simulink model "Rozmyty_adaptacyjny"  (R2017b)
settings: Solver=ode1  StartTime=0.0  StopTime=10  FixedStep=0.0001  RelTol=1e-3
values from neighbouring files (symbols this model uses):
  Kd_adap = 50    [Dane_rozmyte.m]
  Kde1 = 0.02    [Dane_rozmyte.m]
  Kde2 = 0.05    [Dane_rozmyte.m]
  Ke1 = 1    [Dane_rozmyte.m]
  Ke2 = 1    [Dane_rozmyte.m]
  Kp_adap = 750    [Dane_rozmyte.m]
  ksi = 1    [Dane_rozmyte.m]
  Ku1 = 70    [Dane_rozmyte.m]
  Ku2 = 125    [Dane_rozmyte.m]
  omega = 30    [Dane_rozmyte.m]
  Te = 0.001    [Dane_rozmyte.m]
  Tm = 0.2    [Dane_rozmyte.m]
libraries: fuzblock x48
settings Model: Creator=kamil  LastModifiedBy=kamil

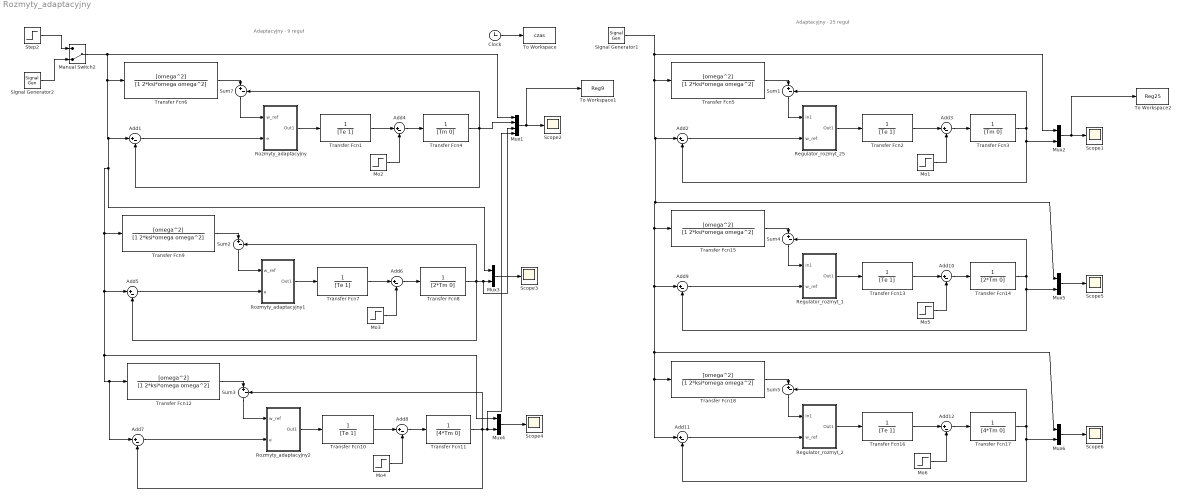
== system Rozmyty_adaptacyjny ==
  note: Adaptacyjny - 9 reguł
  note: Adaptacyjny - 25 reguł
  Add{1..12} (12 alike) : Sum  Inputs=|+-
  Clock : Clock
  Manual Switch2 : ManualSwitch  CurrentSetting=0
  Mo1 : Step  Time=3.5  After=0.5  SampleTime=0
  Mo2 : Step  Time=3  After=0.5  SampleTime=0
  Mo3 : Step  Time=3  After=0.5  SampleTime=0
  Mo4 : Step  Time=3  After=0.5  SampleTime=0
  Mo5 : Step  Time=3.5  After=0.5  SampleTime=0
  Mo6 : Step  Time=3.5  After=0.5  SampleTime=0
  Mux1 : Mux
  Mux{2..6} (5 alike) : Mux  Inputs=2
  Regulator_rozmyt_1 : Subsystem
  Regulator_rozmyt_2 : Subsystem
  Regulator_rozmyt_25 : Subsystem
  Rozmyty_adaptacyjny : Subsystem
  Rozmyty_adaptacyjny1 : Subsystem
  Rozmyty_adaptacyjny2 : Subsystem
  Scope{1..6} (6 alike) : Scope
  Signal Generator1 : SignalGenerator  WaveForm=square  Amplitude=0.25  Frequency=0.25
  Signal Generator2 : SignalGenerator  WaveForm=square  Amplitude=0.25  Frequency=0.25
  Step2 : Step  After=0.25  SampleTime=0
  Sum{1..5,7} (6 alike) : Sum  Inputs=|+-
  To Workspace : ToWorkspace  VariableName=czas  SampleTime=-1
  To Workspace1 : ToWorkspace  VariableName=Reg9  SampleTime=-1
  To Workspace2 : ToWorkspace  VariableName=Reg25  SampleTime=-1
  Transfer Fcn{1..2,7,10,13,16} (6 alike) : TransferFcn  Denominator=[Te 1]
  Transfer Fcn11 : TransferFcn  Denominator=[4*Tm 0]
  Transfer Fcn{5..6,9,12,15,18} (6 alike) : TransferFcn  Numerator=[omega^2]  Denominator=[1 2*ksi*omega omega^2]
  Transfer Fcn14 : TransferFcn  Denominator=[2*Tm 0]
  Transfer Fcn17 : TransferFcn  Denominator=[4*Tm 0]
  Transfer Fcn3 : TransferFcn  Denominator=[Tm 0]
  Transfer Fcn4 : TransferFcn  Denominator=[Tm 0]
  Transfer Fcn8 : TransferFcn  Denominator=[2*Tm 0]
  wires:
  Mo2/1 -> Add4/2
  Add4/1 -> Transfer Fcn4/1
  Transfer Fcn1/1 -> Add4/1
  Add1/1 -> Rozmyty_adaptacyjny/2(e)
  Transfer Fcn4/1 -> Sum7/2, Mux1/2, Add1/2
  Step2/1 -> Manual Switch2/1
  Signal Generator2/1 -> Manual Switch2/2
  Rozmyty_adaptacyjny/1(Out1) -> Transfer Fcn1/1
  Mux1/1 -> To Workspace1/1, Scope2/1
  Sum7/1 -> Rozmyty_adaptacyjny/1(w_ref)
  Transfer Fcn6/1 -> Sum7/1
  Clock/1 -> To Workspace/1
  Regulator_rozmyt_25/1(Out1) -> Transfer Fcn2/1
  Mo1/1 -> Add3/2
  Add3/1 -> Transfer Fcn3/1
  Transfer Fcn3/1 -> Mux2/2, Add2/2, Sum1/2
  Transfer Fcn2/1 -> Add3/1
  Sum1/1 -> Regulator_rozmyt_25/1(In1)
  Mux2/1 -> To Workspace2/1, Scope1/1
  Transfer Fcn5/1 -> Sum1/1
  Add2/1 -> Regulator_rozmyt_25/2(w_ref)
  Sum2/1 -> Rozmyty_adaptacyjny1/1(w_ref)
  Mux3/1 -> Scope3/1
  Transfer Fcn8/1 -> Sum2/2, Mux1/3, Mux3/2, Add5/2
  Transfer Fcn9/1 -> Sum2/1
  Mo3/1 -> Add6/2
  Add5/1 -> Rozmyty_adaptacyjny1/2(e)
  Add6/1 -> Transfer Fcn8/1
  Rozmyty_adaptacyjny1/1(Out1) -> Transfer Fcn7/1
  Transfer Fcn7/1 -> Add6/1
  Sum3/1 -> Rozmyty_adaptacyjny2/1(w_ref)
  Mux4/1 -> Scope4/1
  Transfer Fcn11/1 -> Sum3/2, Mux1/4, Mux4/2, Add7/2
  Transfer Fcn12/1 -> Sum3/1
  Manual Switch2/1 -> Transfer Fcn6/1, Transfer Fcn9/1, Mux4/1, Transfer Fcn12/1, Add7/1, Add5/1, Mux3/1, Add1/1, Mux1/1
  Mo4/1 -> Add8/2
  Add7/1 -> Rozmyty_adaptacyjny2/2(e)
  Add8/1 -> Transfer Fcn11/1
  Rozmyty_adaptacyjny2/1(Out1) -> Transfer Fcn10/1
  Transfer Fcn10/1 -> Add8/1
  Mux5/1 -> Scope5/1
  Add9/1 -> Regulator_rozmyt_1/2(w_ref)
  Transfer Fcn15/1 -> Sum4/1
  Transfer Fcn13/1 -> Add10/1
  Mo5/1 -> Add10/2
  Transfer Fcn14/1 -> Mux5/2, Add9/2, Sum4/2
  Add10/1 -> Transfer Fcn14/1
  Regulator_rozmyt_1/1(Out1) -> Transfer Fcn13/1
  Sum4/1 -> Regulator_rozmyt_1/1(In1)
  Signal Generator1/1 -> Transfer Fcn5/1, Transfer Fcn15/1, Transfer Fcn18/1, Add11/1, Mux6/1, Add9/1, Mux5/1, Add2/1, Mux2/1
  Mux6/1 -> Scope6/1
  Add11/1 -> Regulator_rozmyt_2/2(w_ref)
  Transfer Fcn18/1 -> Sum5/1
  Transfer Fcn16/1 -> Add12/1
  Mo6/1 -> Add12/2
  Transfer Fcn17/1 -> Mux6/2, Add11/2, Sum5/2
  Add12/1 -> Transfer Fcn17/1
  Regulator_rozmyt_2/1(Out1) -> Transfer Fcn16/1
  Sum5/1 -> Regulator_rozmyt_2/1(In1)

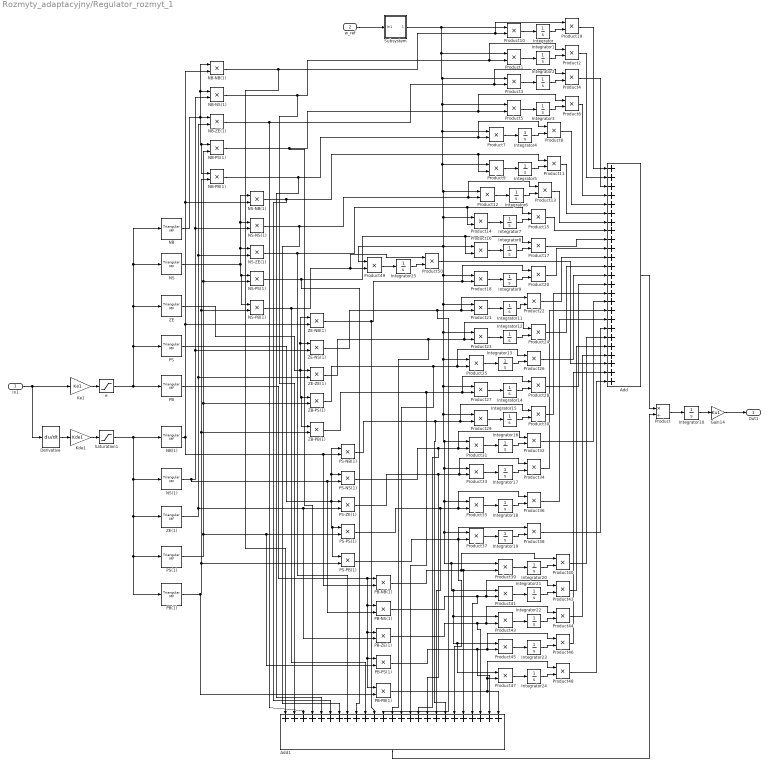
== system Rozmyty_adaptacyjny/Regulator_rozmyt_1 ==
  In1 : Inport
  w_ref : Inport  Port=2
  Add : Sum  Inputs=+++++++++++++++++++++++++
  Add1 : Sum  Inputs=+++++++++++++++++++++++++
  Derivative : Derivative
  Gain14 : Gain  Gain=Ku1
  Integrator{,1..25} (26 alike) : Integrator
  Kde1 : Gain  Gain=Kde1
  Ke1 : Gain  Gain=Ke1
  NB : fuzblock/Membership  Functions/Triangular MF  a=-1.5  b=-1  c=-0.5
      settings: SourceProductName=Fuzzy Logic Toolbox  SourceProductBaseCode=FL
  NB(1) : fuzblock/Membership  Functions/Triangular MF  a=-1.5  b=-1  c=-0.5
      settings: SourceProductName=Fuzzy Logic Toolbox  SourceProductBaseCode=FL
  NB-NB(1) : Product
  NB-NS(1) : Product
  NB-PB(1) : Product
  NB-PS(1) : Product
  NB-ZE(1) : Product
  NS : fuzblock/Membership  Functions/Triangular MF  a=-1  b=-0.5  c=0
      settings: SourceProductName=Fuzzy Logic Toolbox  SourceProductBaseCode=FL
  NS(1) : fuzblock/Membership  Functions/Triangular MF  a=-1  b=-0.5  c=0
      settings: SourceProductName=Fuzzy Logic Toolbox  SourceProductBaseCode=FL
  NS-NB(1) : Product
  NS-NS(1) : Product
  NS-PB(1) : Product
  NS-PS(1) : Product
  NS-ZE(1) : Product
  PB : fuzblock/Membership  Functions/Triangular MF  a=0.5  b=1  c=1.5
      settings: SourceProductName=Fuzzy Logic Toolbox  SourceProductBaseCode=FL
  PB(1) : fuzblock/Membership  Functions/Triangular MF  a=0.5  b=1  c=1.5
      settings: SourceProductName=Fuzzy Logic Toolbox  SourceProductBaseCode=FL
  PB-NB(1) : Product
  PB-NS(1) : Product
  PB-PB(1) : Product
  PB-PS(1) : Product
  PB-ZE(1) : Product
  PS : fuzblock/Membership  Functions/Triangular MF  a=0  b=0.5  c=1
      settings: SourceProductName=Fuzzy Logic Toolbox  SourceProductBaseCode=FL
  PS(1) : fuzblock/Membership  Functions/Triangular MF  a=0  b=0.5  c=1
      settings: SourceProductName=Fuzzy Logic Toolbox  SourceProductBaseCode=FL
  PS-NB(1) : Product
  PS-NS(1) : Product
  PS-PB(1) : Product
  PS-PS(1) : Product
  PS-ZE(1) : Product
  Product : Product  Inputs=*/
  Product{1..50} (50 alike) : Product
  Saturation1 : Saturate  UpperLimit=1  LowerLimit=-1
  Subsystem : Subsystem
  ZB-PB(1) : Product
  ZB-PS(1) : Product
  ZE : fuzblock/Membership  Functions/Triangular MF  a=-0.5  b=0  c=0.5
      settings: SourceProductName=Fuzzy Logic Toolbox  SourceProductBaseCode=FL
  ZE(1) : fuzblock/Membership  Functions/Triangular MF  a=-0.5  b=0  c=0.5
      settings: SourceProductName=Fuzzy Logic Toolbox  SourceProductBaseCode=FL
  ZE-NB(1) : Product
  ZE-NS(1) : Product
  ZE-ZE(1) : Product
  e : Saturate  UpperLimit=1  LowerLimit=-1
  Out1 : Outport
  wires:
  Ke1/1 -> e/1
  Kde1/1 -> Saturation1/1
  Derivative/1 -> Kde1/1
  In1/1 -> Derivative/1, Ke1/1
  e/1 -> PB/1, PS/1, NB/1, NS/1, ZE/1
  Saturation1/1 -> NB(1)/1, NS(1)/1, PB(1)/1, PS(1)/1, ZE(1)/1
  NS/1 -> NS-NB(1)/1, NS-NS(1)/1, NS-ZE(1)/1, NS-PB(1)/1, NS-PS(1)/1
  Add/1 -> Product/1
  Add1/1 -> Product/2
  Integrator10/1 -> Gain14/1
  Product/1 -> Integrator10/1
  Gain14/1 -> Out1/1
  NB/1 -> NB-NB(1)/1, NB-NS(1)/1, NB-ZE(1)/1, NB-PB(1)/1, NB-PS(1)/1
  ZE/1 -> ZE-NB(1)/1, ZE-NS(1)/1, ZE-ZE(1)/1, ZB-PB(1)/1, ZB-PS(1)/1
  PS/1 -> PS-NB(1)/1, PS-NS(1)/1, PS-ZE(1)/1, PS-PB(1)/1, PS-PS(1)/1
  PB/1 -> PB-ZE(1)/1, PB-PB(1)/1, PB-PS(1)/1, PB-NS(1)/1, PB-NB(1)/1
  NB(1)/1 -> PB-NB(1)/2, PS-NB(1)/2, ZE-NB(1)/2, NS-NB(1)/2, NB-NB(1)/2
  NS(1)/1 -> PB-NS(1)/2, PS-NS(1)/2, ZE-NS(1)/2, NS-NS(1)/2, NB-NS(1)/2
  ZE(1)/1 -> PB-ZE(1)/2, PS-ZE(1)/2, ZE-ZE(1)/2, NS-ZE(1)/2, NB-ZE(1)/2
  PS(1)/1 -> PB-PS(1)/2, PS-PS(1)/2, ZB-PS(1)/2, NS-PS(1)/2, NB-PS(1)/2
  PB(1)/1 -> PB-PB(1)/2, PS-PB(1)/2, ZB-PB(1)/2, NS-PB(1)/2, NB-PB(1)/2
  w_ref/1 -> Subsystem/1(In1)
  Product19/1 -> Add/1
  NB-NB(1)/1 -> Add1/1, Product10/2, Product19/1
  Product10/1 -> Integrator/1
  Subsystem/1(Out1) -> Product49/1, Product47/1, Product45/1, Product43/1, Product41/1, Product39/1, Product37/1, Product35/1, Product33/1, Product31/1, Product29/1, Product27/1, Product25/1, Product23/1, Product21/1, Product18/1, Product16/1, Product14/1, Product12/1, Product9/1, Product7/1, Product5/1, Product3/1, Product1/1, Product10/1
  Integrator/1 -> Product19/2
  Integrator1/1 -> Product2/2
  Product1/1 -> Integrator1/1
  NB-NS(1)/1 -> Add1/2, Product2/1, Product1/2
  Product2/1 -> Add/2
  Integrator2/1 -> Product4/2
  Product3/1 -> Integrator2/1
  NB-ZE(1)/1 -> Product4/1, Product3/2, Add1/3
  Product4/1 -> Add/3
  Integrator3/1 -> Product6/2
  Product5/1 -> Integrator3/1
  NB-PS(1)/1 -> Add1/4, Product6/1, Product5/2
  Product6/1 -> Add/4
  Integrator4/1 -> Product8/2
  Product7/1 -> Integrator4/1
  NB-PB(1)/1 -> Add1/5, Product8/1, Product7/2
  Product8/1 -> Add/5
  NS-NB(1)/1 -> Add1/6, Product9/2, Product11/1
  Product9/1 -> Integrator5/1
  Integrator5/1 -> Product11/2
  Product11/1 -> Add/6
  NS-NS(1)/1 -> Add1/7, Product13/1, Product12/2
  Product12/1 -> Integrator6/1
  Integrator6/1 -> Product13/2
  Product13/1 -> Add/7
  NS-ZE(1)/1 -> Add1/8, Product14/2, Product15/1
  Product14/1 -> Integrator7/1
  Integrator7/1 -> Product15/2
  Product15/1 -> Add/8
  NS-PS(1)/1 -> Add1/9, Product16/2, Product17/1
  Product16/1 -> Integrator8/1
  Integrator8/1 -> Product17/2
  Product17/1 -> Add/9
  ZE-NB(1)/1 -> Add1/11, Product18/2, Product20/1
  Product18/1 -> Integrator9/1
  Integrator9/1 -> Product20/2
  Product20/1 -> Add/10
  ZE-NS(1)/1 -> Add1/12, Product22/1, Product21/2
  Product21/1 -> Integrator11/1
  Integrator11/1 -> Product22/2
  Product22/1 -> Add/11
  ZE-ZE(1)/1 -> Add1/13, Product24/1, Product23/2
  Product23/1 -> Integrator12/1
  Integrator12/1 -> Product24/2
  Product24/1 -> Add/12
  ZB-PS(1)/1 -> Add1/14, Product26/1, Product25/2
  Product25/1 -> Integrator13/1
  Integrator13/1 -> Product26/2
  Product26/1 -> Add/13
  ZB-PB(1)/1 -> Add1/15, Product28/1, Product27/2
  Product27/1 -> Integrator14/1
  Integrator14/1 -> Product28/2
  Product28/1 -> Add/14
  PS-NB(1)/1 -> Add1/19, Product29/2, Product30/1
  Product29/1 -> Integrator15/1
  Integrator15/1 -> Product30/2
  PS-NS(1)/1 -> Add1/16, Product32/1, Product31/2
  Product31/1 -> Integrator16/1
  Integrator16/1 -> Product32/2
  PS-ZE(1)/1 -> Add1/17, Product34/1, Product33/2
  Product33/1 -> Integrator17/1
  Integrator17/1 -> Product34/2
  PS-PS(1)/1 -> Add1/18, Product36/1, Product35/2
  Product35/1 -> Integrator18/1
  Integrator18/1 -> Product36/2
  PS-PB(1)/1 -> Add1/20, Product37/2, Product38/1
  Product37/1 -> Integrator19/1
  Integrator19/1 -> Product38/2
  Product39/1 -> Integrator20/1
  Integrator20/1 -> Product40/2
  PB-NB(1)/1 -> Add1/21, Product39/2, Product40/1
  PB-NS(1)/1 -> Add1/22, Product42/1, Product41/2
  Product41/1 -> Integrator21/1
  Integrator21/1 -> Product42/2
  PB-ZE(1)/1 -> Add1/23, Product44/1, Product43/2
  Product43/1 -> Integrator22/1
  Integrator22/1 -> Product44/2
  PB-PS(1)/1 -> Add1/24, Product46/1, Product45/2
  Product45/1 -> Integrator23/1
  Integrator23/1 -> Product46/2
  PB-PB(1)/1 -> Add1/25, Product48/1, Product47/2
  Product47/1 -> Integrator24/1
  Integrator24/1 -> Product48/2
  Product30/1 -> Add/15
  Product32/1 -> Add/16
  Product34/1 -> Add/17
  Product36/1 -> Add/18
  Product38/1 -> Add/19
  Product40/1 -> Add/20
  Product42/1 -> Add/21
  Product44/1 -> Add/22
  Product46/1 -> Add/24
  Product48/1 -> Add/25
  NS-PB(1)/1 -> Add1/10, Product50/1, Product49/2
  Product49/1 -> Integrator25/1
  Integrator25/1 -> Product50/2
  Product50/1 -> Add/23

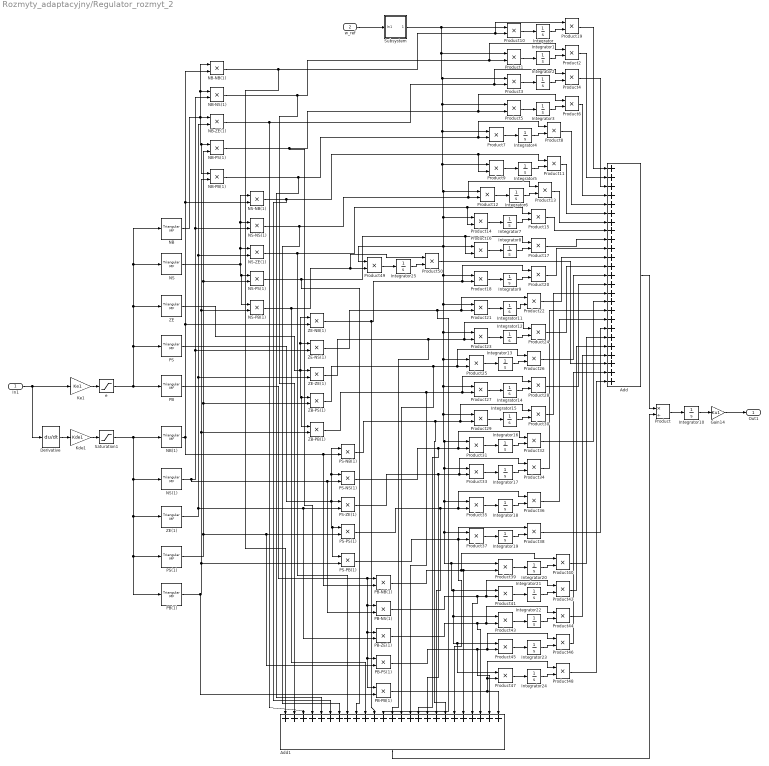
== system Rozmyty_adaptacyjny/Regulator_rozmyt_2 ==
  In1 : Inport
  w_ref : Inport  Port=2
  Add : Sum  Inputs=+++++++++++++++++++++++++
  Add1 : Sum  Inputs=+++++++++++++++++++++++++
  Derivative : Derivative
  Gain14 : Gain  Gain=Ku1
  Integrator{,1..25} (26 alike) : Integrator
  Kde1 : Gain  Gain=Kde1
  Ke1 : Gain  Gain=Ke1
  NB : fuzblock/Membership  Functions/Triangular MF  a=-1.5  b=-1  c=-0.5
      settings: SourceProductName=Fuzzy Logic Toolbox  SourceProductBaseCode=FL
  NB(1) : fuzblock/Membership  Functions/Triangular MF  a=-1.5  b=-1  c=-0.5
      settings: SourceProductName=Fuzzy Logic Toolbox  SourceProductBaseCode=FL
  NB-NB(1) : Product
  NB-NS(1) : Product
  NB-PB(1) : Product
  NB-PS(1) : Product
  NB-ZE(1) : Product
  NS : fuzblock/Membership  Functions/Triangular MF  a=-1  b=-0.5  c=0
      settings: SourceProductName=Fuzzy Logic Toolbox  SourceProductBaseCode=FL
  NS(1) : fuzblock/Membership  Functions/Triangular MF  a=-1  b=-0.5  c=0
      settings: SourceProductName=Fuzzy Logic Toolbox  SourceProductBaseCode=FL
  NS-NB(1) : Product
  NS-NS(1) : Product
  NS-PB(1) : Product
  NS-PS(1) : Product
  NS-ZE(1) : Product
  PB : fuzblock/Membership  Functions/Triangular MF  a=0.5  b=1  c=1.5
      settings: SourceProductName=Fuzzy Logic Toolbox  SourceProductBaseCode=FL
  PB(1) : fuzblock/Membership  Functions/Triangular MF  a=0.5  b=1  c=1.5
      settings: SourceProductName=Fuzzy Logic Toolbox  SourceProductBaseCode=FL
  PB-NB(1) : Product
  PB-NS(1) : Product
  PB-PB(1) : Product
  PB-PS(1) : Product
  PB-ZE(1) : Product
  PS : fuzblock/Membership  Functions/Triangular MF  a=0  b=0.5  c=1
      settings: SourceProductName=Fuzzy Logic Toolbox  SourceProductBaseCode=FL
  PS(1) : fuzblock/Membership  Functions/Triangular MF  a=0  b=0.5  c=1
      settings: SourceProductName=Fuzzy Logic Toolbox  SourceProductBaseCode=FL
  PS-NB(1) : Product
  PS-NS(1) : Product
  PS-PB(1) : Product
  PS-PS(1) : Product
  PS-ZE(1) : Product
  Product : Product  Inputs=*/
  Product{1..50} (50 alike) : Product
  Saturation1 : Saturate  UpperLimit=1  LowerLimit=-1
  Subsystem : Subsystem
  ZB-PB(1) : Product
  ZB-PS(1) : Product
  ZE : fuzblock/Membership  Functions/Triangular MF  a=-0.5  b=0  c=0.5
      settings: SourceProductName=Fuzzy Logic Toolbox  SourceProductBaseCode=FL
  ZE(1) : fuzblock/Membership  Functions/Triangular MF  a=-0.5  b=0  c=0.5
      settings: SourceProductName=Fuzzy Logic Toolbox  SourceProductBaseCode=FL
  ZE-NB(1) : Product
  ZE-NS(1) : Product
  ZE-ZE(1) : Product
  e : Saturate  UpperLimit=1  LowerLimit=-1
  Out1 : Outport
  wires:
  Ke1/1 -> e/1
  Kde1/1 -> Saturation1/1
  Derivative/1 -> Kde1/1
  In1/1 -> Derivative/1, Ke1/1
  e/1 -> PB/1, PS/1, NB/1, NS/1, ZE/1
  Saturation1/1 -> NB(1)/1, NS(1)/1, PB(1)/1, PS(1)/1, ZE(1)/1
  NS/1 -> NS-NB(1)/1, NS-NS(1)/1, NS-ZE(1)/1, NS-PB(1)/1, NS-PS(1)/1
  Add/1 -> Product/1
  Add1/1 -> Product/2
  Integrator10/1 -> Gain14/1
  Product/1 -> Integrator10/1
  Gain14/1 -> Out1/1
  NB/1 -> NB-NB(1)/1, NB-NS(1)/1, NB-ZE(1)/1, NB-PB(1)/1, NB-PS(1)/1
  ZE/1 -> ZE-NB(1)/1, ZE-NS(1)/1, ZE-ZE(1)/1, ZB-PB(1)/1, ZB-PS(1)/1
  PS/1 -> PS-NB(1)/1, PS-NS(1)/1, PS-ZE(1)/1, PS-PB(1)/1, PS-PS(1)/1
  PB/1 -> PB-ZE(1)/1, PB-PB(1)/1, PB-PS(1)/1, PB-NS(1)/1, PB-NB(1)/1
  NB(1)/1 -> PB-NB(1)/2, PS-NB(1)/2, ZE-NB(1)/2, NS-NB(1)/2, NB-NB(1)/2
  NS(1)/1 -> PB-NS(1)/2, PS-NS(1)/2, ZE-NS(1)/2, NS-NS(1)/2, NB-NS(1)/2
  ZE(1)/1 -> PB-ZE(1)/2, PS-ZE(1)/2, ZE-ZE(1)/2, NS-ZE(1)/2, NB-ZE(1)/2
  PS(1)/1 -> PB-PS(1)/2, PS-PS(1)/2, ZB-PS(1)/2, NS-PS(1)/2, NB-PS(1)/2
  PB(1)/1 -> PB-PB(1)/2, PS-PB(1)/2, ZB-PB(1)/2, NS-PB(1)/2, NB-PB(1)/2
  w_ref/1 -> Subsystem/1(In1)
  Product19/1 -> Add/1
  NB-NB(1)/1 -> Add1/1, Product10/2, Product19/1
  Product10/1 -> Integrator/1
  Subsystem/1(Out1) -> Product49/1, Product47/1, Product45/1, Product43/1, Product41/1, Product39/1, Product37/1, Product35/1, Product33/1, Product31/1, Product29/1, Product27/1, Product25/1, Product23/1, Product21/1, Product18/1, Product16/1, Product14/1, Product12/1, Product9/1, Product7/1, Product5/1, Product3/1, Product1/1, Product10/1
  Integrator/1 -> Product19/2
  Integrator1/1 -> Product2/2
  Product1/1 -> Integrator1/1
  NB-NS(1)/1 -> Add1/2, Product2/1, Product1/2
  Product2/1 -> Add/2
  Integrator2/1 -> Product4/2
  Product3/1 -> Integrator2/1
  NB-ZE(1)/1 -> Product4/1, Product3/2, Add1/3
  Product4/1 -> Add/3
  Integrator3/1 -> Product6/2
  Product5/1 -> Integrator3/1
  NB-PS(1)/1 -> Add1/4, Product6/1, Product5/2
  Product6/1 -> Add/4
  Integrator4/1 -> Product8/2
  Product7/1 -> Integrator4/1
  NB-PB(1)/1 -> Add1/5, Product8/1, Product7/2
  Product8/1 -> Add/5
  NS-NB(1)/1 -> Add1/6, Product9/2, Product11/1
  Product9/1 -> Integrator5/1
  Integrator5/1 -> Product11/2
  Product11/1 -> Add/6
  NS-NS(1)/1 -> Add1/7, Product13/1, Product12/2
  Product12/1 -> Integrator6/1
  Integrator6/1 -> Product13/2
  Product13/1 -> Add/7
  NS-ZE(1)/1 -> Add1/8, Product14/2, Product15/1
  Product14/1 -> Integrator7/1
  Integrator7/1 -> Product15/2
  Product15/1 -> Add/8
  NS-PS(1)/1 -> Add1/9, Product16/2, Product17/1
  Product16/1 -> Integrator8/1
  Integrator8/1 -> Product17/2
  Product17/1 -> Add/9
  ZE-NB(1)/1 -> Add1/11, Product18/2, Product20/1
  Product18/1 -> Integrator9/1
  Integrator9/1 -> Product20/2
  Product20/1 -> Add/10
  ZE-NS(1)/1 -> Add1/12, Product22/1, Product21/2
  Product21/1 -> Integrator11/1
  Integrator11/1 -> Product22/2
  Product22/1 -> Add/11
  ZE-ZE(1)/1 -> Add1/13, Product24/1, Product23/2
  Product23/1 -> Integrator12/1
  Integrator12/1 -> Product24/2
  Product24/1 -> Add/12
  ZB-PS(1)/1 -> Add1/14, Product26/1, Product25/2
  Product25/1 -> Integrator13/1
  Integrator13/1 -> Product26/2
  Product26/1 -> Add/13
  ZB-PB(1)/1 -> Add1/15, Product28/1, Product27/2
  Product27/1 -> Integrator14/1
  Integrator14/1 -> Product28/2
  Product28/1 -> Add/14
  PS-NB(1)/1 -> Add1/19, Product29/2, Product30/1
  Product29/1 -> Integrator15/1
  Integrator15/1 -> Product30/2
  PS-NS(1)/1 -> Add1/16, Product32/1, Product31/2
  Product31/1 -> Integrator16/1
  Integrator16/1 -> Product32/2
  PS-ZE(1)/1 -> Add1/17, Product34/1, Product33/2
  Product33/1 -> Integrator17/1
  Integrator17/1 -> Product34/2
  PS-PS(1)/1 -> Add1/18, Product36/1, Product35/2
  Product35/1 -> Integrator18/1
  Integrator18/1 -> Product36/2
  PS-PB(1)/1 -> Add1/20, Product37/2, Product38/1
  Product37/1 -> Integrator19/1
  Integrator19/1 -> Product38/2
  Product39/1 -> Integrator20/1
  Integrator20/1 -> Product40/2
  PB-NB(1)/1 -> Add1/21, Product39/2, Product40/1
  PB-NS(1)/1 -> Add1/22, Product42/1, Product41/2
  Product41/1 -> Integrator21/1
  Integrator21/1 -> Product42/2
  PB-ZE(1)/1 -> Add1/23, Product44/1, Product43/2
  Product43/1 -> Integrator22/1
  Integrator22/1 -> Product44/2
  PB-PS(1)/1 -> Add1/24, Product46/1, Product45/2
  Product45/1 -> Integrator23/1
  Integrator23/1 -> Product46/2
  PB-PB(1)/1 -> Add1/25, Product48/1, Product47/2
  Product47/1 -> Integrator24/1
  Integrator24/1 -> Product48/2
  Product30/1 -> Add/15
  Product32/1 -> Add/16
  Product34/1 -> Add/17
  Product36/1 -> Add/18
  Product38/1 -> Add/19
  Product40/1 -> Add/20
  Product42/1 -> Add/21
  Product44/1 -> Add/22
  Product46/1 -> Add/24
  Product48/1 -> Add/25
  NS-PB(1)/1 -> Add1/10, Product50/1, Product49/2
  Product49/1 -> Integrator25/1
  Integrator25/1 -> Product50/2
  Product50/1 -> Add/23

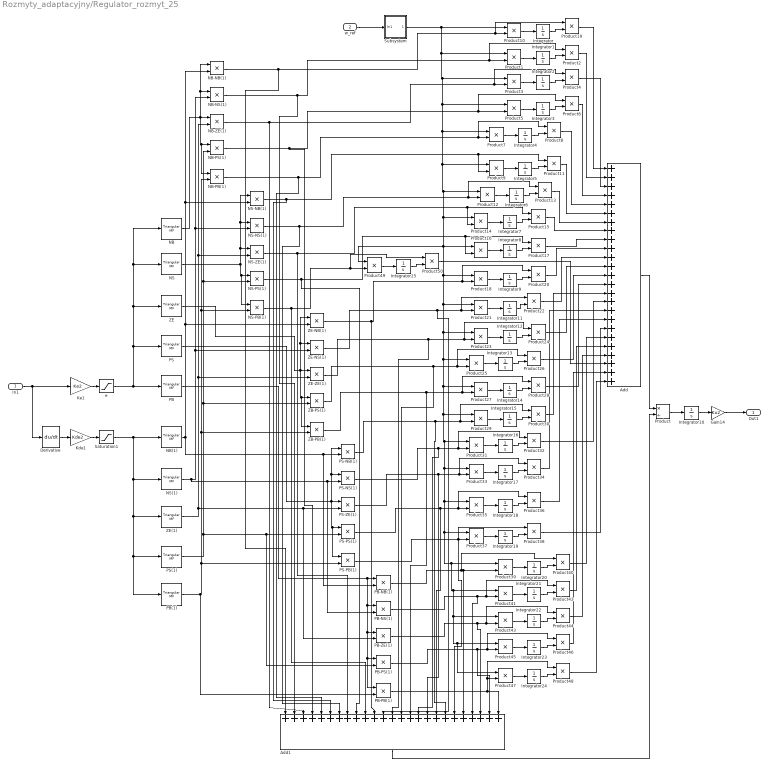
== system Rozmyty_adaptacyjny/Regulator_rozmyt_25 ==
  In1 : Inport
  w_ref : Inport  Port=2
  Add : Sum  Inputs=+++++++++++++++++++++++++
  Add1 : Sum  Inputs=+++++++++++++++++++++++++
  Derivative : Derivative
  Gain14 : Gain  Gain=Ku2
  Integrator{,1..25} (26 alike) : Integrator
  Kde1 : Gain  Gain=Kde2
  Ke1 : Gain  Gain=Ke2
  NB : fuzblock/Membership  Functions/Triangular MF  a=-1.5  b=-1  c=-0.5
      settings: SourceProductName=Fuzzy Logic Toolbox  SourceProductBaseCode=FL
  NB(1) : fuzblock/Membership  Functions/Triangular MF  a=-1.5  b=-1  c=-0.5
      settings: SourceProductName=Fuzzy Logic Toolbox  SourceProductBaseCode=FL
  NB-NB(1) : Product
  NB-NS(1) : Product
  NB-PB(1) : Product
  NB-PS(1) : Product
  NB-ZE(1) : Product
  NS : fuzblock/Membership  Functions/Triangular MF  a=-1  b=-0.5  c=0
      settings: SourceProductName=Fuzzy Logic Toolbox  SourceProductBaseCode=FL
  NS(1) : fuzblock/Membership  Functions/Triangular MF  a=-1  b=-0.5  c=0
      settings: SourceProductName=Fuzzy Logic Toolbox  SourceProductBaseCode=FL
  NS-NB(1) : Product
  NS-NS(1) : Product
  NS-PB(1) : Product
  NS-PS(1) : Product
  NS-ZE(1) : Product
  PB : fuzblock/Membership  Functions/Triangular MF  a=0.5  b=1  c=1.5
      settings: SourceProductName=Fuzzy Logic Toolbox  SourceProductBaseCode=FL
  PB(1) : fuzblock/Membership  Functions/Triangular MF  a=0.5  b=1  c=1.5
      settings: SourceProductName=Fuzzy Logic Toolbox  SourceProductBaseCode=FL
  PB-NB(1) : Product
  PB-NS(1) : Product
  PB-PB(1) : Product
  PB-PS(1) : Product
  PB-ZE(1) : Product
  PS : fuzblock/Membership  Functions/Triangular MF  a=0  b=0.5  c=1
      settings: SourceProductName=Fuzzy Logic Toolbox  SourceProductBaseCode=FL
  PS(1) : fuzblock/Membership  Functions/Triangular MF  a=0  b=0.5  c=1
      settings: SourceProductName=Fuzzy Logic Toolbox  SourceProductBaseCode=FL
  PS-NB(1) : Product
  PS-NS(1) : Product
  PS-PB(1) : Product
  PS-PS(1) : Product
  PS-ZE(1) : Product
  Product : Product  Inputs=*/
  Product{1..50} (50 alike) : Product
  Saturation1 : Saturate  UpperLimit=1  LowerLimit=-1
  Subsystem : Subsystem
  ZB-PB(1) : Product
  ZB-PS(1) : Product
  ZE : fuzblock/Membership  Functions/Triangular MF  a=-0.5  b=0  c=0.5
      settings: SourceProductName=Fuzzy Logic Toolbox  SourceProductBaseCode=FL
  ZE(1) : fuzblock/Membership  Functions/Triangular MF  a=-0.5  b=0  c=0.5
      settings: SourceProductName=Fuzzy Logic Toolbox  SourceProductBaseCode=FL
  ZE-NB(1) : Product
  ZE-NS(1) : Product
  ZE-ZE(1) : Product
  e : Saturate  UpperLimit=1  LowerLimit=-1
  Out1 : Outport
  wires:
  Ke1/1 -> e/1
  Kde1/1 -> Saturation1/1
  Derivative/1 -> Kde1/1
  In1/1 -> Derivative/1, Ke1/1
  e/1 -> PB/1, PS/1, NB/1, NS/1, ZE/1
  Saturation1/1 -> NB(1)/1, NS(1)/1, PB(1)/1, PS(1)/1, ZE(1)/1
  NS/1 -> NS-NB(1)/1, NS-NS(1)/1, NS-ZE(1)/1, NS-PB(1)/1, NS-PS(1)/1
  Add/1 -> Product/1
  Add1/1 -> Product/2
  Integrator10/1 -> Gain14/1
  Product/1 -> Integrator10/1
  Gain14/1 -> Out1/1
  NB/1 -> NB-NB(1)/1, NB-NS(1)/1, NB-ZE(1)/1, NB-PB(1)/1, NB-PS(1)/1
  ZE/1 -> ZE-NB(1)/1, ZE-NS(1)/1, ZE-ZE(1)/1, ZB-PB(1)/1, ZB-PS(1)/1
  PS/1 -> PS-NB(1)/1, PS-NS(1)/1, PS-ZE(1)/1, PS-PB(1)/1, PS-PS(1)/1
  PB/1 -> PB-ZE(1)/1, PB-PB(1)/1, PB-PS(1)/1, PB-NS(1)/1, PB-NB(1)/1
  NB(1)/1 -> PB-NB(1)/2, PS-NB(1)/2, ZE-NB(1)/2, NS-NB(1)/2, NB-NB(1)/2
  NS(1)/1 -> PB-NS(1)/2, PS-NS(1)/2, ZE-NS(1)/2, NS-NS(1)/2, NB-NS(1)/2
  ZE(1)/1 -> PB-ZE(1)/2, PS-ZE(1)/2, ZE-ZE(1)/2, NS-ZE(1)/2, NB-ZE(1)/2
  PS(1)/1 -> PB-PS(1)/2, PS-PS(1)/2, ZB-PS(1)/2, NS-PS(1)/2, NB-PS(1)/2
  PB(1)/1 -> PB-PB(1)/2, PS-PB(1)/2, ZB-PB(1)/2, NS-PB(1)/2, NB-PB(1)/2
  w_ref/1 -> Subsystem/1(In1)
  Product19/1 -> Add/1
  NB-NB(1)/1 -> Add1/1, Product10/2, Product19/1
  Product10/1 -> Integrator/1
  Subsystem/1(Out1) -> Product49/1, Product47/1, Product45/1, Product43/1, Product41/1, Product39/1, Product37/1, Product35/1, Product33/1, Product31/1, Product29/1, Product27/1, Product25/1, Product23/1, Product21/1, Product18/1, Product16/1, Product14/1, Product12/1, Product9/1, Product7/1, Product5/1, Product3/1, Product1/1, Product10/1
  Integrator/1 -> Product19/2
  Integrator1/1 -> Product2/2
  Product1/1 -> Integrator1/1
  NB-NS(1)/1 -> Add1/2, Product2/1, Product1/2
  Product2/1 -> Add/2
  Integrator2/1 -> Product4/2
  Product3/1 -> Integrator2/1
  NB-ZE(1)/1 -> Product4/1, Product3/2, Add1/3
  Product4/1 -> Add/3
  Integrator3/1 -> Product6/2
  Product5/1 -> Integrator3/1
  NB-PS(1)/1 -> Add1/4, Product6/1, Product5/2
  Product6/1 -> Add/4
  Integrator4/1 -> Product8/2
  Product7/1 -> Integrator4/1
  NB-PB(1)/1 -> Add1/5, Product8/1, Product7/2
  Product8/1 -> Add/5
  NS-NB(1)/1 -> Add1/6, Product9/2, Product11/1
  Product9/1 -> Integrator5/1
  Integrator5/1 -> Product11/2
  Product11/1 -> Add/6
  NS-NS(1)/1 -> Add1/7, Product13/1, Product12/2
  Product12/1 -> Integrator6/1
  Integrator6/1 -> Product13/2
  Product13/1 -> Add/7
  NS-ZE(1)/1 -> Add1/8, Product14/2, Product15/1
  Product14/1 -> Integrator7/1
  Integrator7/1 -> Product15/2
  Product15/1 -> Add/8
  NS-PS(1)/1 -> Add1/9, Product16/2, Product17/1
  Product16/1 -> Integrator8/1
  Integrator8/1 -> Product17/2
  Product17/1 -> Add/9
  ZE-NB(1)/1 -> Add1/11, Product18/2, Product20/1
  Product18/1 -> Integrator9/1
  Integrator9/1 -> Product20/2
  Product20/1 -> Add/10
  ZE-NS(1)/1 -> Add1/12, Product22/1, Product21/2
  Product21/1 -> Integrator11/1
  Integrator11/1 -> Product22/2
  Product22/1 -> Add/11
  ZE-ZE(1)/1 -> Add1/13, Product24/1, Product23/2
  Product23/1 -> Integrator12/1
  Integrator12/1 -> Product24/2
  Product24/1 -> Add/12
  ZB-PS(1)/1 -> Add1/14, Product26/1, Product25/2
  Product25/1 -> Integrator13/1
  Integrator13/1 -> Product26/2
  Product26/1 -> Add/13
  ZB-PB(1)/1 -> Add1/15, Product28/1, Product27/2
  Product27/1 -> Integrator14/1
  Integrator14/1 -> Product28/2
  Product28/1 -> Add/14
  PS-NB(1)/1 -> Add1/19, Product29/2, Product30/1
  Product29/1 -> Integrator15/1
  Integrator15/1 -> Product30/2
  PS-NS(1)/1 -> Add1/16, Product32/1, Product31/2
  Product31/1 -> Integrator16/1
  Integrator16/1 -> Product32/2
  PS-ZE(1)/1 -> Add1/17, Product34/1, Product33/2
  Product33/1 -> Integrator17/1
  Integrator17/1 -> Product34/2
  PS-PS(1)/1 -> Add1/18, Product36/1, Product35/2
  Product35/1 -> Integrator18/1
  Integrator18/1 -> Product36/2
  PS-PB(1)/1 -> Add1/20, Product37/2, Product38/1
  Product37/1 -> Integrator19/1
  Integrator19/1 -> Product38/2
  Product39/1 -> Integrator20/1
  Integrator20/1 -> Product40/2
  PB-NB(1)/1 -> Add1/21, Product39/2, Product40/1
  PB-NS(1)/1 -> Add1/22, Product42/1, Product41/2
  Product41/1 -> Integrator21/1
  Integrator21/1 -> Product42/2
  PB-ZE(1)/1 -> Add1/23, Product44/1, Product43/2
  Product43/1 -> Integrator22/1
  Integrator22/1 -> Product44/2
  PB-PS(1)/1 -> Add1/24, Product46/1, Product45/2
  Product45/1 -> Integrator23/1
  Integrator23/1 -> Product46/2
  PB-PB(1)/1 -> Add1/25, Product48/1, Product47/2
  Product47/1 -> Integrator24/1
  Integrator24/1 -> Product48/2
  Product30/1 -> Add/15
  Product32/1 -> Add/16
  Product34/1 -> Add/17
  Product36/1 -> Add/18
  Product38/1 -> Add/19
  Product40/1 -> Add/20
  Product42/1 -> Add/21
  Product44/1 -> Add/22
  Product46/1 -> Add/24
  Product48/1 -> Add/25
  NS-PB(1)/1 -> Add1/10, Product50/1, Product49/2
  Product49/1 -> Integrator25/1
  Integrator25/1 -> Product50/2
  Product50/1 -> Add/23

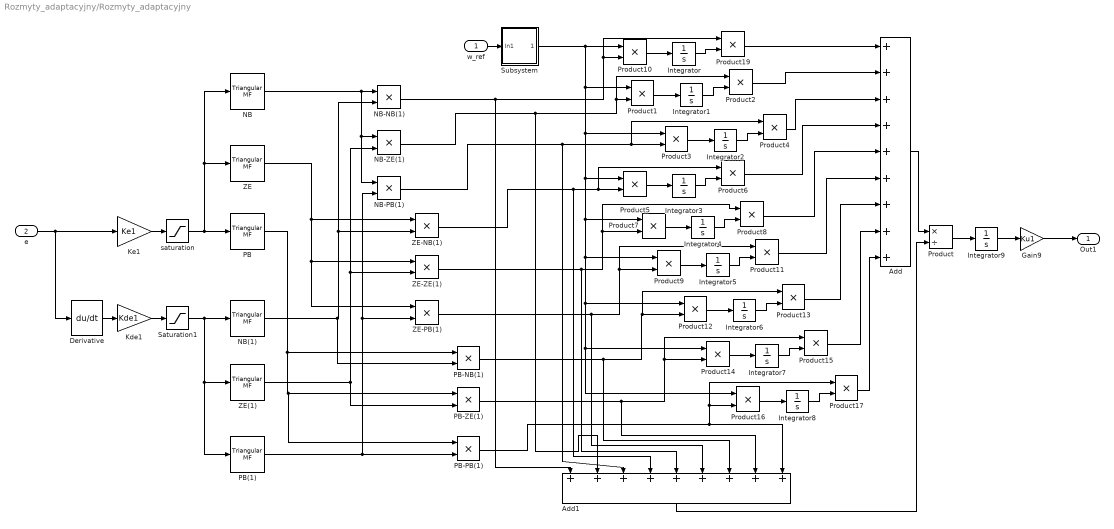
== system Rozmyty_adaptacyjny/Rozmyty_adaptacyjny ==
  w_ref : Inport
  e : Inport  Port=2
  Add : Sum  Inputs=+++++++++
  Add1 : Sum  Inputs=+++++++++
  Derivative : Derivative
  Gain9 : Gain  Gain=Ku1
  Integrator{,1..9} (10 alike) : Integrator
  Kde1 : Gain  Gain=Kde1
  Ke1 : Gain  Gain=Ke1
  NB : fuzblock/Membership  Functions/Triangular MF  a=-2  b=-1  c=0
      settings: SourceProductName=Fuzzy Logic Toolbox  SourceProductBaseCode=FL
  NB(1) : fuzblock/Membership  Functions/Triangular MF  a=-2  b=-1  c=0
      settings: SourceProductName=Fuzzy Logic Toolbox  SourceProductBaseCode=FL
  NB-NB(1) : Product
  NB-PB(1) : Product
  NB-ZE(1) : Product
  PB : fuzblock/Membership  Functions/Triangular MF  a=0  b=1  c=2
      settings: SourceProductName=Fuzzy Logic Toolbox  SourceProductBaseCode=FL
  PB(1) : fuzblock/Membership  Functions/Triangular MF  a=0  b=1  c=2
      settings: SourceProductName=Fuzzy Logic Toolbox  SourceProductBaseCode=FL
  PB-NB(1) : Product
  PB-PB(1) : Product
  PB-ZE(1) : Product
  Product : Product  Inputs=*/
  Product{1..17,19} (18 alike) : Product
  Saturation1 : Saturate  UpperLimit=1  LowerLimit=-1
  Subsystem : Subsystem
  ZE : fuzblock/Membership  Functions/Triangular MF  a=-1  b=0  c=1
      settings: SourceProductName=Fuzzy Logic Toolbox  SourceProductBaseCode=FL
  ZE(1) : fuzblock/Membership  Functions/Triangular MF  a=-1  b=0  c=1
      settings: SourceProductName=Fuzzy Logic Toolbox  SourceProductBaseCode=FL
  ZE-NB(1) : Product
  ZE-PB(1) : Product
  ZE-ZE(1) : Product
  saturation : Saturate  UpperLimit=1  LowerLimit=-1
  Out1 : Outport
  wires:
  Ke1/1 -> saturation/1
  Kde1/1 -> Saturation1/1
  Derivative/1 -> Kde1/1
  e/1 -> Derivative/1, Ke1/1
  saturation/1 -> PB/1, NB/1, ZE/1
  Saturation1/1 -> PB(1)/1, ZE(1)/1, NB(1)/1
  NB/1 -> NB-ZE(1)/1, NB-PB(1)/1, NB-NB(1)/1
  NB(1)/1 -> PB-NB(1)/2, NB-NB(1)/2, ZE-NB(1)/2
  ZE(1)/1 -> PB-ZE(1)/2, NB-ZE(1)/2, ZE-ZE(1)/2
  PB(1)/1 -> NB-PB(1)/2, ZE-PB(1)/2, PB-PB(1)/2
  ZE/1 -> ZE-NB(1)/1, ZE-ZE(1)/1, ZE-PB(1)/1
  PB/1 -> PB-NB(1)/1, PB-PB(1)/1, PB-ZE(1)/1
  Add/1 -> Product/1
  Add1/1 -> Product/2
  Integrator9/1 -> Gain9/1
  Product/1 -> Integrator9/1
  Gain9/1 -> Out1/1
  Product10/1 -> Integrator/1
  Integrator/1 -> Product19/2
  Product19/1 -> Add/1
  w_ref/1 -> Subsystem/1(In1)
  Product1/1 -> Integrator1/1
  NB-ZE(1)/1 -> Add1/2, Product1/2, Product2/1
  NB-NB(1)/1 -> Product10/2, Product19/1, Add1/1
  Integrator1/1 -> Product2/2
  Product2/1 -> Add/2
  Product3/1 -> Integrator2/1
  NB-PB(1)/1 -> Add1/3, Product4/1, Product3/2
  Integrator2/1 -> Product4/2
  Product4/1 -> Add/3
  Product5/1 -> Integrator3/1
  ZE-NB(1)/1 -> Add1/4, Product6/1, Product5/2
  Integrator3/1 -> Product6/2
  Product6/1 -> Add/4
  Product7/1 -> Integrator4/1
  ZE-ZE(1)/1 -> Add1/5, Product7/2, Product8/1
  Integrator4/1 -> Product8/2
  Product8/1 -> Add/5
  Product9/1 -> Integrator5/1
  ZE-PB(1)/1 -> Add1/6, Product11/1, Product9/2
  Integrator5/1 -> Product11/2
  Product11/1 -> Add/6
  Product12/1 -> Integrator6/1
  PB-NB(1)/1 -> Add1/7, Product13/1, Product12/2
  Integrator6/1 -> Product13/2
  Product13/1 -> Add/7
  Product14/1 -> Integrator7/1
  PB-ZE(1)/1 -> Product15/1, Product14/2, Add1/8
  Integrator7/1 -> Product15/2
  Product15/1 -> Add/8
  Product16/1 -> Integrator8/1
  PB-PB(1)/1 -> Add1/9, Product17/1, Product16/2
  Subsystem/1(Out1) -> Product5/1, Product16/1, Product14/1, Product12/1, Product9/1, Product7/1, Product3/1, Product1/1, Product10/1
  Integrator8/1 -> Product17/2
  Product17/1 -> Add/9

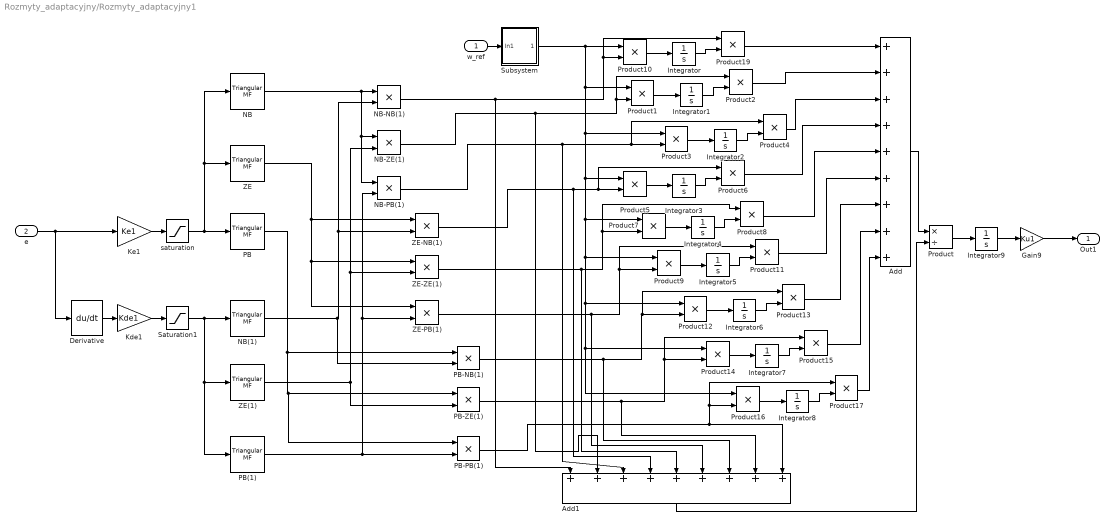
== system Rozmyty_adaptacyjny/Rozmyty_adaptacyjny1 ==
  w_ref : Inport
  e : Inport  Port=2
  Add : Sum  Inputs=+++++++++
  Add1 : Sum  Inputs=+++++++++
  Derivative : Derivative
  Gain9 : Gain  Gain=Ku1
  Integrator{,1..9} (10 alike) : Integrator
  Kde1 : Gain  Gain=Kde1
  Ke1 : Gain  Gain=Ke1
  NB : fuzblock/Membership  Functions/Triangular MF  a=-2  b=-1  c=0
      settings: SourceProductName=Fuzzy Logic Toolbox  SourceProductBaseCode=FL
  NB(1) : fuzblock/Membership  Functions/Triangular MF  a=-2  b=-1  c=0
      settings: SourceProductName=Fuzzy Logic Toolbox  SourceProductBaseCode=FL
  NB-NB(1) : Product
  NB-PB(1) : Product
  NB-ZE(1) : Product
  PB : fuzblock/Membership  Functions/Triangular MF  a=0  b=1  c=2
      settings: SourceProductName=Fuzzy Logic Toolbox  SourceProductBaseCode=FL
  PB(1) : fuzblock/Membership  Functions/Triangular MF  a=0  b=1  c=2
      settings: SourceProductName=Fuzzy Logic Toolbox  SourceProductBaseCode=FL
  PB-NB(1) : Product
  PB-PB(1) : Product
  PB-ZE(1) : Product
  Product : Product  Inputs=*/
  Product{1..17,19} (18 alike) : Product
  Saturation1 : Saturate  UpperLimit=1  LowerLimit=-1
  Subsystem : Subsystem
  ZE : fuzblock/Membership  Functions/Triangular MF  a=-1  b=0  c=1
      settings: SourceProductName=Fuzzy Logic Toolbox  SourceProductBaseCode=FL
  ZE(1) : fuzblock/Membership  Functions/Triangular MF  a=-1  b=0  c=1
      settings: SourceProductName=Fuzzy Logic Toolbox  SourceProductBaseCode=FL
  ZE-NB(1) : Product
  ZE-PB(1) : Product
  ZE-ZE(1) : Product
  saturation : Saturate  UpperLimit=1  LowerLimit=-1
  Out1 : Outport
  wires:
  Ke1/1 -> saturation/1
  Kde1/1 -> Saturation1/1
  Derivative/1 -> Kde1/1
  e/1 -> Derivative/1, Ke1/1
  saturation/1 -> PB/1, NB/1, ZE/1
  Saturation1/1 -> PB(1)/1, ZE(1)/1, NB(1)/1
  NB/1 -> NB-ZE(1)/1, NB-PB(1)/1, NB-NB(1)/1
  NB(1)/1 -> PB-NB(1)/2, NB-NB(1)/2, ZE-NB(1)/2
  ZE(1)/1 -> PB-ZE(1)/2, NB-ZE(1)/2, ZE-ZE(1)/2
  PB(1)/1 -> NB-PB(1)/2, ZE-PB(1)/2, PB-PB(1)/2
  ZE/1 -> ZE-NB(1)/1, ZE-ZE(1)/1, ZE-PB(1)/1
  PB/1 -> PB-NB(1)/1, PB-PB(1)/1, PB-ZE(1)/1
  Add/1 -> Product/1
  Add1/1 -> Product/2
  Integrator9/1 -> Gain9/1
  Product/1 -> Integrator9/1
  Gain9/1 -> Out1/1
  Product10/1 -> Integrator/1
  Integrator/1 -> Product19/2
  Product19/1 -> Add/1
  w_ref/1 -> Subsystem/1(In1)
  Product1/1 -> Integrator1/1
  NB-ZE(1)/1 -> Add1/2, Product1/2, Product2/1
  NB-NB(1)/1 -> Product10/2, Product19/1, Add1/1
  Integrator1/1 -> Product2/2
  Product2/1 -> Add/2
  Product3/1 -> Integrator2/1
  NB-PB(1)/1 -> Add1/3, Product4/1, Product3/2
  Integrator2/1 -> Product4/2
  Product4/1 -> Add/3
  Product5/1 -> Integrator3/1
  ZE-NB(1)/1 -> Add1/4, Product6/1, Product5/2
  Integrator3/1 -> Product6/2
  Product6/1 -> Add/4
  Product7/1 -> Integrator4/1
  ZE-ZE(1)/1 -> Add1/5, Product7/2, Product8/1
  Integrator4/1 -> Product8/2
  Product8/1 -> Add/5
  Product9/1 -> Integrator5/1
  ZE-PB(1)/1 -> Add1/6, Product11/1, Product9/2
  Integrator5/1 -> Product11/2
  Product11/1 -> Add/6
  Product12/1 -> Integrator6/1
  PB-NB(1)/1 -> Add1/7, Product13/1, Product12/2
  Integrator6/1 -> Product13/2
  Product13/1 -> Add/7
  Product14/1 -> Integrator7/1
  PB-ZE(1)/1 -> Product15/1, Product14/2, Add1/8
  Integrator7/1 -> Product15/2
  Product15/1 -> Add/8
  Product16/1 -> Integrator8/1
  PB-PB(1)/1 -> Add1/9, Product17/1, Product16/2
  Subsystem/1(Out1) -> Product5/1, Product16/1, Product14/1, Product12/1, Product9/1, Product7/1, Product3/1, Product1/1, Product10/1
  Integrator8/1 -> Product17/2
  Product17/1 -> Add/9

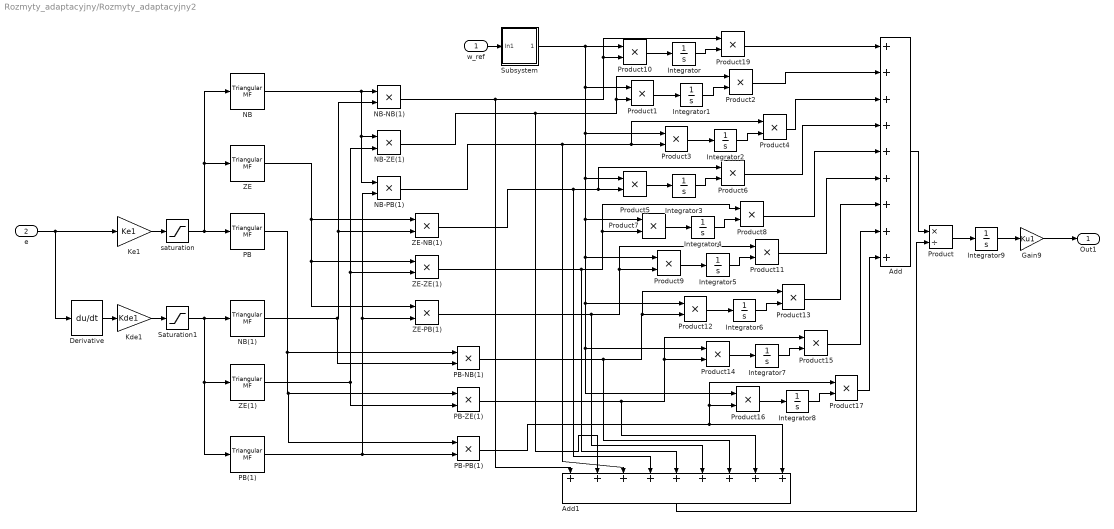
== system Rozmyty_adaptacyjny/Rozmyty_adaptacyjny2 ==
  w_ref : Inport
  e : Inport  Port=2
  Add : Sum  Inputs=+++++++++
  Add1 : Sum  Inputs=+++++++++
  Derivative : Derivative
  Gain9 : Gain  Gain=Ku1
  Integrator{,1..9} (10 alike) : Integrator
  Kde1 : Gain  Gain=Kde1
  Ke1 : Gain  Gain=Ke1
  NB : fuzblock/Membership  Functions/Triangular MF  a=-2  b=-1  c=0
      settings: SourceProductName=Fuzzy Logic Toolbox  SourceProductBaseCode=FL
  NB(1) : fuzblock/Membership  Functions/Triangular MF  a=-2  b=-1  c=0
      settings: SourceProductName=Fuzzy Logic Toolbox  SourceProductBaseCode=FL
  NB-NB(1) : Product
  NB-PB(1) : Product
  NB-ZE(1) : Product
  PB : fuzblock/Membership  Functions/Triangular MF  a=0  b=1  c=2
      settings: SourceProductName=Fuzzy Logic Toolbox  SourceProductBaseCode=FL
  PB(1) : fuzblock/Membership  Functions/Triangular MF  a=0  b=1  c=2
      settings: SourceProductName=Fuzzy Logic Toolbox  SourceProductBaseCode=FL
  PB-NB(1) : Product
  PB-PB(1) : Product
  PB-ZE(1) : Product
  Product : Product  Inputs=*/
  Product{1..17,19} (18 alike) : Product
  Saturation1 : Saturate  UpperLimit=1  LowerLimit=-1
  Subsystem : Subsystem
  ZE : fuzblock/Membership  Functions/Triangular MF  a=-1  b=0  c=1
      settings: SourceProductName=Fuzzy Logic Toolbox  SourceProductBaseCode=FL
  ZE(1) : fuzblock/Membership  Functions/Triangular MF  a=-1  b=0  c=1
      settings: SourceProductName=Fuzzy Logic Toolbox  SourceProductBaseCode=FL
  ZE-NB(1) : Product
  ZE-PB(1) : Product
  ZE-ZE(1) : Product
  saturation : Saturate  UpperLimit=1  LowerLimit=-1
  Out1 : Outport
  wires:
  Ke1/1 -> saturation/1
  Kde1/1 -> Saturation1/1
  Derivative/1 -> Kde1/1
  e/1 -> Derivative/1, Ke1/1
  saturation/1 -> PB/1, NB/1, ZE/1
  Saturation1/1 -> PB(1)/1, ZE(1)/1, NB(1)/1
  NB/1 -> NB-ZE(1)/1, NB-PB(1)/1, NB-NB(1)/1
  NB(1)/1 -> PB-NB(1)/2, NB-NB(1)/2, ZE-NB(1)/2
  ZE(1)/1 -> PB-ZE(1)/2, NB-ZE(1)/2, ZE-ZE(1)/2
  PB(1)/1 -> NB-PB(1)/2, ZE-PB(1)/2, PB-PB(1)/2
  ZE/1 -> ZE-NB(1)/1, ZE-ZE(1)/1, ZE-PB(1)/1
  PB/1 -> PB-NB(1)/1, PB-PB(1)/1, PB-ZE(1)/1
  Add/1 -> Product/1
  Add1/1 -> Product/2
  Integrator9/1 -> Gain9/1
  Product/1 -> Integrator9/1
  Gain9/1 -> Out1/1
  Product10/1 -> Integrator/1
  Integrator/1 -> Product19/2
  Product19/1 -> Add/1
  w_ref/1 -> Subsystem/1(In1)
  Product1/1 -> Integrator1/1
  NB-ZE(1)/1 -> Add1/2, Product1/2, Product2/1
  NB-NB(1)/1 -> Product10/2, Product19/1, Add1/1
  Integrator1/1 -> Product2/2
  Product2/1 -> Add/2
  Product3/1 -> Integrator2/1
  NB-PB(1)/1 -> Add1/3, Product4/1, Product3/2
  Integrator2/1 -> Product4/2
  Product4/1 -> Add/3
  Product5/1 -> Integrator3/1
  ZE-NB(1)/1 -> Add1/4, Product6/1, Product5/2
  Integrator3/1 -> Product6/2
  Product6/1 -> Add/4
  Product7/1 -> Integrator4/1
  ZE-ZE(1)/1 -> Add1/5, Product7/2, Product8/1
  Integrator4/1 -> Product8/2
  Product8/1 -> Add/5
  Product9/1 -> Integrator5/1
  ZE-PB(1)/1 -> Add1/6, Product11/1, Product9/2
  Integrator5/1 -> Product11/2
  Product11/1 -> Add/6
  Product12/1 -> Integrator6/1
  PB-NB(1)/1 -> Add1/7, Product13/1, Product12/2
  Integrator6/1 -> Product13/2
  Product13/1 -> Add/7
  Product14/1 -> Integrator7/1
  PB-ZE(1)/1 -> Product15/1, Product14/2, Add1/8
  Integrator7/1 -> Product15/2
  Product15/1 -> Add/8
  Product16/1 -> Integrator8/1
  PB-PB(1)/1 -> Add1/9, Product17/1, Product16/2
  Subsystem/1(Out1) -> Product5/1, Product16/1, Product14/1, Product12/1, Product9/1, Product7/1, Product3/1, Product1/1, Product10/1
  Integrator8/1 -> Product17/2
  Product17/1 -> Add/9

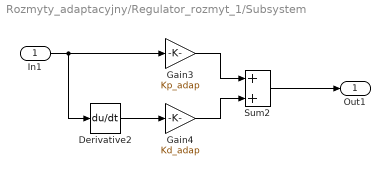
== system Rozmyty_adaptacyjny/Regulator_rozmyt_1/Subsystem ==
  In1 : Inport
  Derivative2 : Derivative
  Gain3 : Gain  Gain=Kp_adap
  Gain4 : Gain  Gain=Kd_adap
  Sum2 : Sum
  Out1 : Outport
  wires:
  Derivative2/1 -> Gain4/1
  Gain3/1 -> Sum2/1
  In1/1 -> Derivative2/1, Gain3/1
  Sum2/1 -> Out1/1
  Gain4/1 -> Sum2/2

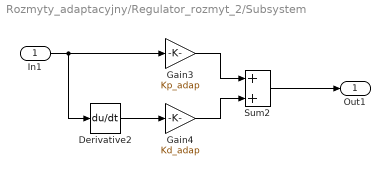
== system Rozmyty_adaptacyjny/Regulator_rozmyt_2/Subsystem ==
  In1 : Inport
  Derivative2 : Derivative
  Gain3 : Gain  Gain=Kp_adap
  Gain4 : Gain  Gain=Kd_adap
  Sum2 : Sum
  Out1 : Outport
  wires:
  Derivative2/1 -> Gain4/1
  Gain3/1 -> Sum2/1
  In1/1 -> Derivative2/1, Gain3/1
  Sum2/1 -> Out1/1
  Gain4/1 -> Sum2/2

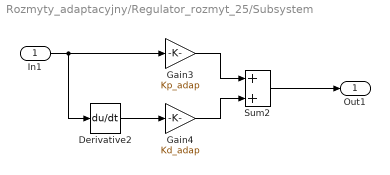
== system Rozmyty_adaptacyjny/Regulator_rozmyt_25/Subsystem ==
  In1 : Inport
  Derivative2 : Derivative
  Gain3 : Gain  Gain=Kp_adap
  Gain4 : Gain  Gain=Kd_adap
  Sum2 : Sum
  Out1 : Outport
  wires:
  Derivative2/1 -> Gain4/1
  Gain3/1 -> Sum2/1
  In1/1 -> Derivative2/1, Gain3/1
  Sum2/1 -> Out1/1
  Gain4/1 -> Sum2/2

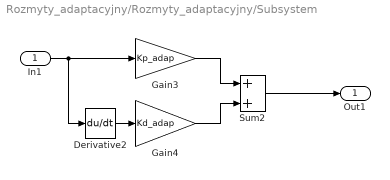
== system Rozmyty_adaptacyjny/Rozmyty_adaptacyjny/Subsystem ==
  In1 : Inport
  Derivative2 : Derivative
  Gain3 : Gain  Gain=Kp_adap
  Gain4 : Gain  Gain=Kd_adap
  Sum2 : Sum
  Out1 : Outport
  wires:
  Derivative2/1 -> Gain4/1
  Gain3/1 -> Sum2/1
  In1/1 -> Derivative2/1, Gain3/1
  Sum2/1 -> Out1/1
  Gain4/1 -> Sum2/2

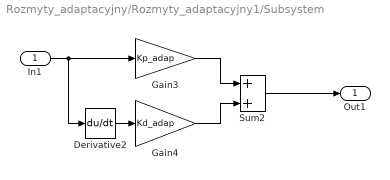
== system Rozmyty_adaptacyjny/Rozmyty_adaptacyjny1/Subsystem ==
  In1 : Inport
  Derivative2 : Derivative
  Gain3 : Gain  Gain=Kp_adap
  Gain4 : Gain  Gain=Kd_adap
  Sum2 : Sum
  Out1 : Outport
  wires:
  Derivative2/1 -> Gain4/1
  Gain3/1 -> Sum2/1
  In1/1 -> Derivative2/1, Gain3/1
  Sum2/1 -> Out1/1
  Gain4/1 -> Sum2/2

== system Rozmyty_adaptacyjny/Rozmyty_adaptacyjny2/Subsystem ==
  In1 : Inport
  Derivative2 : Derivative
  Gain3 : Gain  Gain=Kp_adap
  Gain4 : Gain  Gain=Kd_adap
  Sum2 : Sum
  Out1 : Outport
  wires:
  Derivative2/1 -> Gain4/1
  Gain3/1 -> Sum2/1
  In1/1 -> Derivative2/1, Gain3/1
  Sum2/1 -> Out1/1
  Gain4/1 -> Sum2/2
